simulink model "FYP_Model_OpenLoop"  (R2014b)
settings: Solver=ode3  StartTime=0.0  StopTime=5  FixedStep=0.00001  MaxStep=0.00001  MinStep=0.00002  RelTol=1e-3
values from neighbouring files (symbols this model uses):
  C = 2.2389314028e-09    [Example_Data.mat]    (also in calculate_constants.m = sqrt(I*K)/Q)
  I = 2.138022e-10    [Example_Data.mat]    (also in calculate_constants.m = (1/12)*m*w*w)
  K = 8.44057253633e-05    [Example_Data.mat]    (also in calculate_constants.m = Wn*Wn*I)
  theta = [-7.61408173959 -7.51775010326 -7.42143983606 -7.32515065184 -7.22888226498 -7.13263439042 -7.03640674362 -6.94019904057 -6.84401099779 -6.74784233231 -6.65169276165 -6.55556200382 ... (160 elements, 1x160)]    [Example_Data.mat]    (also in SC_Transformation.m = (asin(x1/3000))*(180/pi))
  TorqueN = [1.05331979874e-12 9.29651153439e-13 1.4049471593e-12 1.07667428419e-12 1.24916097602e-12 1.30962949594e-12 1.37528218875e-12 1.44578522446e-12 1.52178717406e-12 1.6037356104e-12 1.6116506126e-12 1.87151628256e-12 ... (160 elements, 1x160)]    [Example_Data.mat]    (also in SC_Transformation.m = Torque/(V*V))
  V = 60    [Example_Data.mat]    (also in SC_Transformation.m = 30; Simulink_Iterate.m = V_array(i))
libraries: simulink x4
settings Model: Creator=Kishan  LastModifiedBy=Kishan
settings DataIOCC: SaveFormat=StructureWithTime  SaveOutput=off  ReturnWorkspaceOutputsName=yout

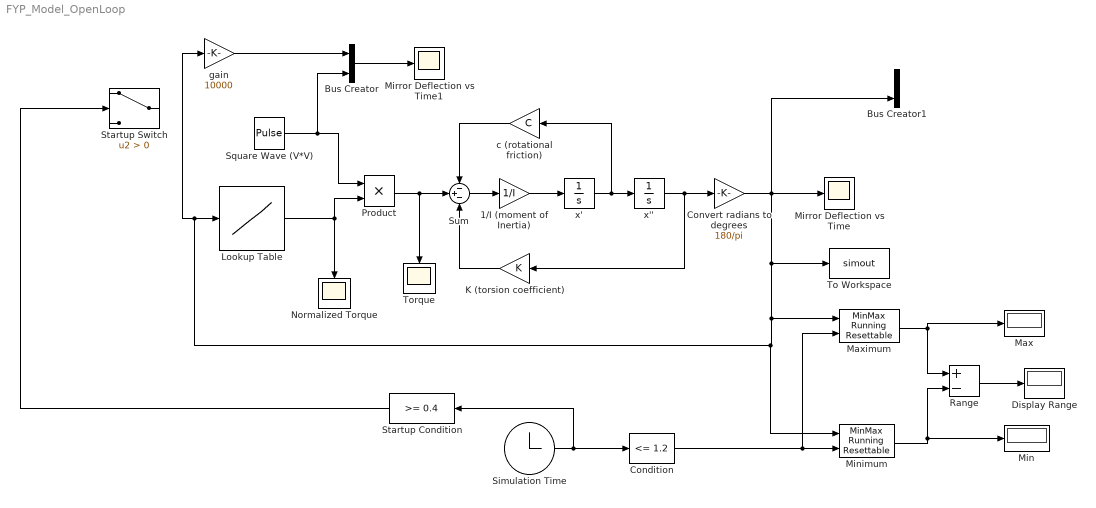
== system FYP_Model_OpenLoop ==
  "       K (torsion coefficient)" : Gain  Gain=K
  1/I (moment of Inertia) : Gain  Gain=1/I
  Bus Creator : BusCreator  Inputs=2
  Bus Creator1 : BusCreator  Inputs=2
  Condition : simulink/Logic and Bit Operations/Compare To Constant  relop=<=  const=1.2  OutDataTypeStr=boolean
  Convert radians to degrees : Gain  Gain=180/pi
  Display Range : Display
  Lookup Table : Lookup_n-D  NumberOfTableDimensions=1  BreakpointsForDimension1=theta  IndexSearchMethod=Linear search  Table=TorqueN  InternalRulePriority=Speed  RndMeth=Simplest  InputSameDT=on
  Max : Display
  Maximum : simulink/Math Operations/MinMax Running Resettable  Function=max  vinit=0.0
  Min : Display
  Minimum : simulink/Math Operations/MinMax Running Resettable  Function=min  vinit=10
  Mirror Deflection vs Time : Scope
      settings: TimeRange=1.5
  Mirror Deflection vs Time1 : Scope
      settings: TimeRange=1.5  YMin=-2000  YMax=4000  SaveName=ScopeData2
  Normalized Torque : Scope
      settings: TimeRange=0.009043223963749458  YMin=0  YMax=1
  Product : Product
  Range : Sum  Inputs=+-
  Simulation Time : Clock
  Square Wave (V*V) : DiscretePulseGenerator  PulseType=Time based  Amplitude=V*V  Period=0.0049  PulseWidth=20  SampleTime=0.0025
  Startup Condition : simulink/Logic and Bit Operations/Compare To Constant  relop=>=  const=0.4  OutDataTypeStr=uint8
  Startup Switch : Switch  Criteria=u2 > Threshold
  Sum : Sum  Inputs=-+-
  To Workspace : ToWorkspace  VariableName=simout  SaveFormat=Structure With Time  SampleTime=-1
  Torque : Scope
      settings: TimeRange=0.009043223963749458  YMin=0  YMax=1  SaveName=ScopeData3
  c (rotational friction) : Gain  Gain=C
  gain : Gain  Gain=10000
  x' : Integrator
  x'' : Integrator
  wires:
  x'/1 -> x''/1, c (rotational friction)/1
  1/I (moment of Inertia)/1 -> x'/1
  Sum/1 -> 1/I (moment of Inertia)/1
  "       K (torsion coefficient)"/1 -> Sum/3
  c (rotational friction)/1 -> Sum/1
  Lookup Table/1 -> Product/2, Normalized Torque/1
  Product/1 -> Torque/1, Sum/2
  x''/1 -> Convert radians to degrees/1, "       K (torsion coefficient)"/1
  Bus Creator/1 -> Mirror Deflection vs Time1/1
  gain/1 -> Bus Creator/1
  Minimum/1 -> Min/1, Range/2
  Maximum/1 -> Max/1, Range/1
  Range/1 -> Display Range/1
  Condition/1 -> Maximum/2, Minimum/2
  Convert radians to degrees/1 -> Bus Creator1/2, To Workspace/1, Maximum/1, Minimum/1, gain/1, Lookup Table/1, Mirror Deflection vs Time/1
  Simulation Time/1 -> Startup Condition/1, Condition/1
  Startup Condition/1 -> Startup Switch/2
  ? -> Startup Switch/3
  ? -> Startup Switch/1
  Square Wave (V*V)/1 -> Bus Creator/2, Product/1
